simulink model "Controle_Adaptativo_PPR"  (R2024b)
settings: Solver=FixedStepAuto  StartTime=0.0  StopTime=5  FixedStep=0.01  RelTol=1e-3
InitFcn:
  | clear
  | %Massa
  | m1 = 1;
  | m2 = 2;
  | m3 = 1.5;
  | g = 9.81;
  | L3 = 1.2;
  | I3 = 0.01;
  | 
  | %Estimativa Inicial da massa
  | Pi = [m1+m2+m3;m2+m3;m3*L3;I3+m3*L3^2];
  | 
  | %Massa Estimadas
  | m1 = 1.2;
  | m2 = 1.8;
  | m3 = 1.2;
  | g = 9.81;
  | L3 = 1;
  | I3 = 0.005;
  | 
  | %Estimativa Inicial da massa
  | pih0 = [m1+m2+m3;m2+m3;m3*L3;I3+m3*L3^2];
  | 
  | %Parâmetros do Controlador PD
  | Kp = 100;
  | Kd = 50*eye(3);
  | 
  | %Parâmetros da Lei de Aprendizagem
  | Gamma = 100*eye(4);
  | 
  | %Parâmetro da filtragem do erro
  | Lambda = 100*eye(3);
StopFcn:
  | syms d1 d2 real
  | tdh_n =[0 pi/2 d1 pi/2;
  |                0 pi/2 d2 pi/2];
  | info = [2;2];
  | q = out.logsout{1}.Values.Data;
  | tout = out.tout;
  | for i =1:length(tout)
  |     zd(i,1) = out.logsout{1}.Values.Data(1,1,i);
  |     xd(i,1) = out.logsout{1}.Values.Data(2,1,i);
  |     q1(i,1) = out.logsout{3}.Values.Data(1,1,i);
  |     q2(i,1) = out.logsout{3}.Values.Data(2,1,i);
  | end
  | ref = [xd zeros(length(tout),1) zd];
  | qout = [q1 q2];
  | 
  | dinanima_ref(tdh_n,info,qout,tout,1,ref')
values from neighbouring files (symbols this model uses):
  xd = out.logsout{2}.Values.Data    [anima_simulink.m]
settings Model: Creator=IDRZBOOK002  LastModifiedBy=IDRZBOOK002

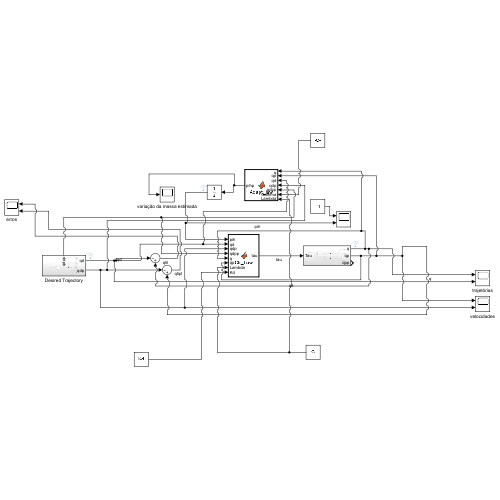
[thumbnail: Simulink's stored preview of the top-level diagram]
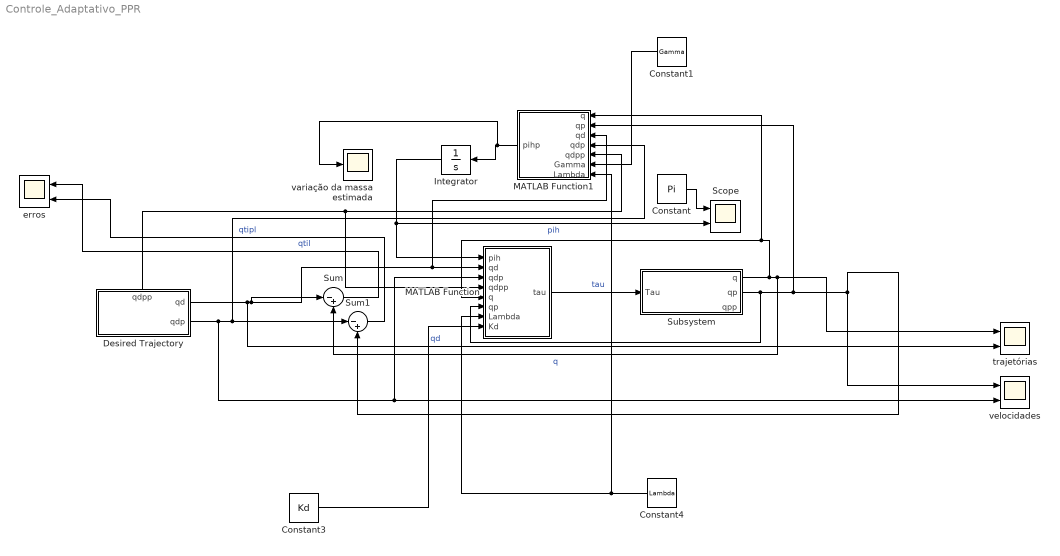
== system Controle_Adaptativo_PPR ==
  Constant : Constant  Value=Pi
  Constant1 : Constant  Value=Gamma
  Constant3 : Constant  Value=Kd
  Constant4 : Constant  Value=Lambda
  Desired Trajectory : Subsystem
      settings: PortSchema="{\"entries\":[{\"content\":{\"sides\":[{\"content\":{},\"type\":\"ConnectorPlacement.EquallySpacedRectSide\",\"uuid\":\"fde9c678-b2f0-48bb-8b77-059617d4abcd\"},{\"content\":{\"connectorIds\":[\"Out1\",\"Out2\"],\"side\":\"RIGHT\"},\"type\":\"ConnectorPlacement.EquallySpacedRectSide\",\"uuid\":\"217a379d-a803-41b8-8b57-bfab0073b449\"},{\"content\":{\"connectorIds\":[\"Out3\"],\"side\":\"TOP\"},\"type\":\"ConnectorPlacement.EquallySpacedRectSide\",\"uuid\":\"f11199d7-3a24-4232-8e20-31e0b008a8a8\"}]},\"type\":\"ConnectorPlacement.EquallySpacedConnector\",\"uuid\":\"b1296899-b312-4960-bb2e-673c4701805b\"}],\"packageUris\":[\"http://schema.mathworks.com/mf0/Connector/R2020b\"],\"version\":\"1.0\"}"
  Integrator : Integrator  InitialCondition=pih0
  MATLAB Function : MATLAB Function  TreatAsAtomicUnit=on
  MATLAB Function1 : MATLAB Function  TreatAsAtomicUnit=on
  Scope : Scope  NumInputPorts=2
  Subsystem : Subsystem
  Sum : Sum  Inputs=|-+
  Sum1 : Sum  Inputs=|-+
  erros : Scope  NumInputPorts=2
  trajetórias : Scope  NumInputPorts=2
  variação da massa estimada : Scope
  velocidades : Scope  NumInputPorts=2
  wires:
  Desired Trajectory/1(qd) -> MATLAB Function1/3(qd), MATLAB Function/2(qd), Sum/1, trajetórias/2  "qd"
  MATLAB Function/1(tau) -> Subsystem/1(Tau)  "tau"
  Sum/1 -> erros/1  "qtil"
  Sum1/1 -> erros/2  "qtipl"
  Subsystem/1(q) -> MATLAB Function1/1(q), MATLAB Function/5(q), trajetórias/1, Sum/2  "q"
  Subsystem/2(qp) -> MATLAB Function/6(qp), MATLAB Function1/2(qp), velocidades/1, Sum1/2
  Desired Trajectory/2(qdp) -> MATLAB Function/3(qdp), velocidades/2, MATLAB Function1/4(qdp), Sum1/1
  Integrator/1 -> MATLAB Function/1(pih), Scope/2  "pih"
  Constant/1 -> Scope/1
  Constant1/1 -> MATLAB Function1/6(Gamma)
  Constant3/1 -> MATLAB Function/8(Kd)
  Constant4/1 -> MATLAB Function/7(Lambda), MATLAB Function1/7(Lambda)
  Desired Trajectory/3(qdpp) -> MATLAB Function1/5(qdpp), MATLAB Function/4(qdpp)
  MATLAB Function1/1(pihp) -> variação da massa estimada/1, Integrator/1

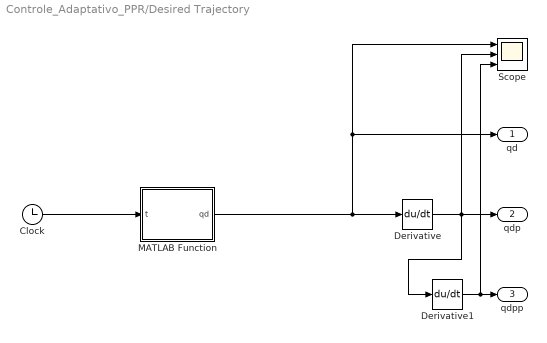
== system Controle_Adaptativo_PPR/Desired Trajectory ==
  Clock : Clock
  Derivative : Derivative
  Derivative1 : Derivative
  MATLAB Function : MATLAB Function  TreatAsAtomicUnit=on
  Scope : Scope  NumInputPorts=3
  qd : Outport
  qdp : Outport  Port=2
  qdpp : Outport  Port=3
  wires:
  Clock/1 -> MATLAB Function/1(t)
  MATLAB Function/1(qd) -> qd/1, Scope/1, Derivative/1
  Derivative/1 -> Scope/2, Derivative1/1, qdp/1
  Derivative1/1 -> Scope/3, qdpp/1

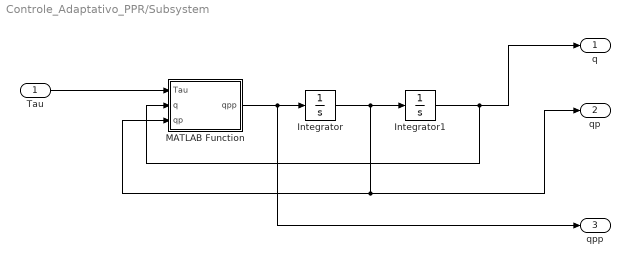
== system Controle_Adaptativo_PPR/Subsystem ==
  Tau : Inport
  Integrator : Integrator
  Integrator1 : Integrator
  MATLAB Function : MATLAB Function  TreatAsAtomicUnit=on
  q : Outport
  qp : Outport  Port=2
  qpp : Outport  Port=3
  wires:
  Tau/1 -> MATLAB Function/1(Tau)
  Integrator/1 -> qp/1, MATLAB Function/3(qp), Integrator1/1
  Integrator1/1 -> MATLAB Function/2(q), q/1
  MATLAB Function/1(qpp) -> qpp/1, Integrator/1

== matlab function Controle_Adaptativo_PPR/MATLAB Function1 ==
  data: q input; qp input; qd input; qdp input; qdpp input; Gamma input; Lambda input; pihp output size=[4 1]
function pihp = Adapt_law(q,qp,qd, qdp,qdpp, Gamma, Lambda)
pihp = zeros(4, 1);
%Variáveis de junta lidas e desejadas
d1pp = qdpp(1);
d2pp = qdpp(2);
thpp = qdpp(3);
d1pd = qdp(1);
d2pd = qdp(2);
thpd = qdp(3);
d1p = qp(1);
d2p = qp(2);
thp = qp(3);
th = q(3);
%Constantes
g = 9.81;
%Matriz Regressora
Y = [d1pp+g 0 -sin(th)*thpp-cos(th)*thp*thpd 0;
    0 d2pp cos(th)*thpp-sin(th)*thp*thpd 0;
    0 0 -sin(th)*d1pp+cos(th)*d2pp-g*sin(th) thpp];
sigma = (qp-qdp) + Lambda * (q-qd);
pihp = -Gamma^-1*Y'*sigma;

== matlab function Controle_Adaptativo_PPR/MATLAB Function ==
  data: pih input; qd input; tau output size=[3 1]; qdp input; qdpp input; q input; qp input; Lambda input; Kd input
function tau = Ctr_Law(pih,qd,qdp,qdpp,q,qp, Lambda, Kd)
%Variáveis de junta lidas e desejadas
d1pp = qdpp(1);
d2pp = qdpp(2);
thpp = qdpp(3);
d1pd = qdp(1);
d2pd = qdp(2);
thpd = qdp(3);
d1p = qp(1);
d2p = qp(2);
thp = qp(3);
th = q(3);
%Constantes
g = 9.81;
%Matriz Regressora
Y = [d1pp+g 0 -sin(th)*thpp-cos(th)*thp*thpd 0;
    0 d2pp cos(th)*thpp-sin(th)*thp*thpd 0;
    0 0 -sin(th)*d1pp+cos(th)*d2pp-g*sin(th) thpp];
sigma = (qp-qdp) + Lambda * (q-qd);
tau = Y*pih-Kd*sigma;

== matlab function Controle_Adaptativo_PPR/Desired Trajectory/MATLAB Function ==
  data: t input; qd output
function qd= traj_des(t)
qd = [sin(2*t)+sin(3*t);cos(2*t)+cos(5*t);0];

== matlab function Controle_Adaptativo_PPR/Subsystem/MATLAB Function ==
  data: Tau input; qpp output; q input; qp input
function qpp = Din(Tau,q,qp)
qpp = zeros(3, 1);
%Variáveis de junta
th = q(3);
dth = qp(3);
%Parâmetros do modelo
m1 = 1;
m2 = 2;
m3 = 1.5;
g = 9.81;
L3 = 1.2;
I3 = 0.01;
%Matrizes da dinâmica
H = [         m1 + m2 + m3,                    0, -0.5000*L3*m3*sin(th);
     0,              m2 + m3,  0.5000*L3*m3*cos(th);
    -0.5000*L3*m3*sin(th), 0.5000*L3*m3*cos(th),   0.2500*m3*L3^2 + I3];
C = [0, 0, -0.5000*L3*dth*m3*cos(th);
0, 0, -0.5000*L3*dth*m3*sin(th);
0, 0,                         0];

G =  [0;g*(m2 + m3);0.5000*L3*g*m3*cos(th)];

%Cálculo da aceleração
qpp = H^-1*(Tau-C*qp-G);
